simulink model "simpleMicrogrid_v3_0_18a"  (R2018a)
settings: Solver=VariableStepAuto  StartTime=0.0  StopTime=30  RelTol=1e-3
undefined symbols (not defined in the file or in its folder): Ion, Lithium
libraries: simulink x21, spsSeriesRLCBranchLib x13, spsIdealSwitchLib x10, spsMosfetLib x8, spsPWMGeneratorDCDCLib x6, spsVoltageMeasurementLib x5, spsThreePhaseSeriesRLCLoadLib x3, spsThreePhaseSeriesRLCBranchLib x3, spsThreePhaseDynamicLoadLib x3, spsGroundLib x2, spsThreePhaseVIMeasurementLib x2, spsUniversalBridgeLib x2
(part 1 of 2)
settings Model: SimulationMode=accelerator  Creator=jakub  LastModifiedBy=mluser
settings DataIOCC: ReturnWorkspaceOutputs=on
settings SFSimCC: SimUseLocalCustomCode=on
settings RTWCC: RTWUseLocalCustomCode=on

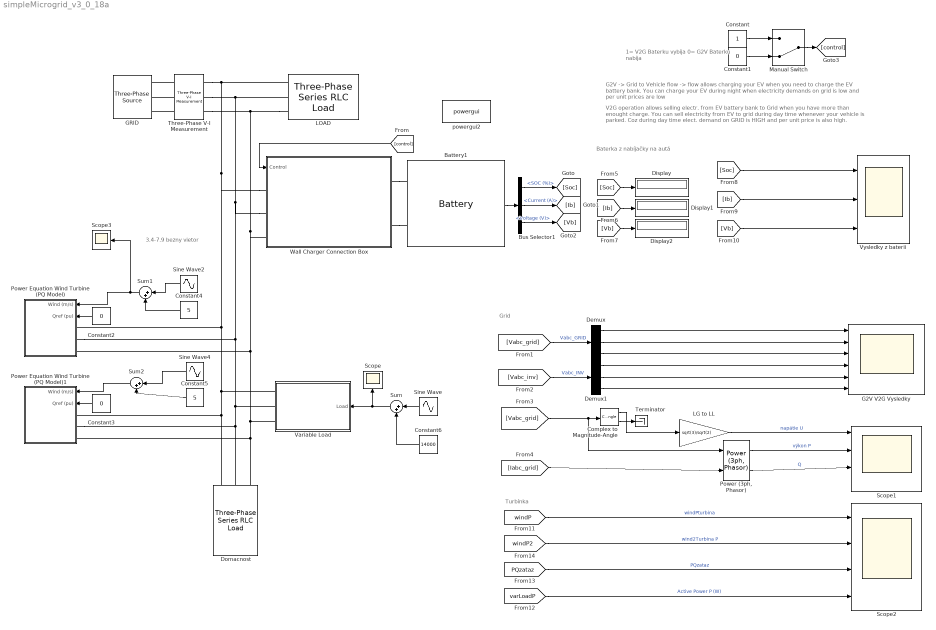
== system simpleMicrogrid_v3_0_18a ==
  note: 3.4-7.9 bezny vietor
  note: Baterka z nabíjačky na autá
  note: Turbínka
  note: Grid
  note: 1= V2G Baterku vybíja
      | 0= G2V Baterku nabíja
  note: G2V -> Grid to Vehicle flow -> flow allows charging your EV when you need to charge the EV battery bank. You can charge your EV during night when electricity demands on grid is low and per unit prices are low
  note: V2G operation allows selling electr. from EV battery bank to Grid when you have more than enought charge. You can sell electricity from EV to grid during day time whenever your vehicle is parked. Coz during day time elect. demand on GRID is HIGH and per unit price is also high.
  Battery1 : spsBatteryLib/Battery  BatType=Lithium-Ion  ShowTempParam=off  ThermalPreset=no  ShowAgeParam=off  NomV=230  NomQ=100  SOC=60  Batt_Tr=1e-3  PresetModel=on  MaxQ=100  MinV=172.5  FullV=267.717  Dis_rate=43.4783  R=0.023  Normal_OP=90.4348  expZone="[248.4887      4.913043]"  current=[6.5 13 32.5]  Units=Time  Tci=20  NomT=20  T2=-30  MaxQ2=4.8  FullV2=7.1  Normal_OP2=5.655  expZone2="[6.58           1]"  Rca=0.6  ti=2000  Dp=0  Neq0=0  Tsim=1e6  Ta1=25  Qeol=5.4*0.9  Reol=0.013333*1.2  Char_age=[2.3478, 3]  Dis_age=[2.3478, 10]  N1=1500  N2=10500  N3=1000  N4=1400  Ta2=45  N5=950
  Bus Selector1 : BusSelector  OutputSignals=SOC (%),Current (A),Voltage (V)
  Complex to Magnitude-Angle : ComplexToMagnitudeAngle
  Constant : Constant
  Constant1 : Constant  Value=0
  Constant2 : Constant  Value=0
  Constant3 : Constant  Value=0
  Constant4 : Constant  Value=5
  Constant5 : Constant  Value=5
  Constant6 : Constant  Value=14000
  Demux : Demux  Outputs=3
  Demux1 : Demux  Outputs=3
  Display : Display
  Display1 : Display
  Display2 : Display
  Domacnost : spsThreePhaseSeriesRLCLoadLib/Three-Phase Series RLC Load  LConnTagsString=A|B|C  Configuration=Y (grounded)  NominalVoltage=380  Vabc=[1e3 1e3 1e3]  Vabcp=[1e3 1e3 1e3]  NominalFrequency=50  UnbalancedPower=off  ActivePower=10e3  InductivePower=0  CapacitivePower=0  Pabc=[10e3 9e3 11e3]  QLabc=[100 90 110]  QCabc=[100 90 110]  Pabcp=[10e3 9e3 11e3]  QLabcp=[100 90 110]  QCabcp=[100 90 110]  Measurements=None  LoadType=constant Z
  G2V V2G Vysledky : Scope  NumInputPorts=6
  GRID : spsThreePhaseSourceLib/Three-Phase Source  InternalConnection=Yg  VoltagePhases=off  Voltage=380  PhaseAngle=0  Voltage_phases=[25e3 25e3 25e3]/sqrt(3)  PhaseAngles_phases=[0 -120 +120]  Frequency=50  NonIdealSource=on  SpecifyImpedance=on  Resistance=0.8929  Inductance=16.58e-3  ShortCircuitLevel=100e6  BaseVoltage=380  XRratio=7  BusType=swing  Pref=10e3  Qref=0  Prefabc=[10e3, 10e3, 10e3]  Qrefabc=[0, 0, 0]  Qmin=-inf  Qmax=inf
  LG to LL : Gain  Gain=sqrt(3)/sqrt(2)
  LOAD : spsThreePhaseSeriesRLCLoadLib/Three-Phase Series RLC Load  LConnTagsString=A|B|C  Configuration=Y (grounded)  NominalVoltage=380  Vabc=[1e3 1e3 1e3]  Vabcp=[1e3 1e3 1e3]  NominalFrequency=50  UnbalancedPower=off  ActivePower=10e3  InductivePower=0  CapacitivePower=0  Pabc=[10e3 9e3 11e3]  QLabc=[100 90 110]  QCabc=[100 90 110]  Pabcp=[10e3 9e3 11e3]  QLabcp=[100 90 110]  QCabcp=[100 90 110]  Measurements=None  LoadType=constant Z
  Manual Switch : ManualSwitch  CurrentSetting=0
  "Power (3ph, Phasor)" : spsPower3phPhasorLib/Power (3ph, Phasor)
      settings: SourceProductBaseCode=PS
  Power Equation Wind Turbine (PQ Model) : Subsystem  AncestorBlock=|  mask{Unom=15, Umax=25, Umin=5, Pselect=Simple Cubic Power, rp=5, Cp=16/27, rho=1.225, Pnom=500e3, Uvec=[1:1:30], Pvec=[0,0,0,0,21359.3750000000,58193.5000000000,104316.125000000,157104.500000000,213935.875000000,272187.500000000,329236.625000000,382460.500000000,429236.375000000,466941.500000000,492953.125000000,500000,500000,500000,500000,500000,500000,500000,500000,500000,500000,0,0,0,0,0], Tp=0.1, Tq=1, ReactP=30}
      | exampleMicrogridLibrary/Power Equation
      | Wind Turbine
      | (PQ Model)
      mask prompts: Unom "Nominal Wind Speed [m/s]"; Umax "Maximum Operating Wind [m/s]"; Umin "Minimum Operating Wind [m/s]"; Pselect "Wind Turbine Power Method"; rp "Blade Radius, r [m]"; Cp "Performance Coefficient, Cp"; rho "Air Density, rho [kg/m^3]"; Pnom "Nominal Power, [W]"; Uvec "Wind Vec [m/s]"; Pvec "Power Vec [W]"; Tp "Active Power Dynamics, Tp [s]"; Tq "Reactive Power Dynamics, Tq [s]"; ReactP "Reactive Power Percentage [%]"
      mask help:
      | Simple Wind Turbine that serves as an Active and Reactive Power Source depending on the Wind Power Curve.
      |
      | The Wind Turbine Power Curve can be defined by:
      | - Dimentions of the wind turbine
      | - Simple cubic power curve
      | - Look-up vector from a wind turbine data sheet.
      mask init:
      | A = pi*rp^2;
      | 
      | if Pselect == 1,
      |     Pmax = 1/2*rho*Cp*A*Umax^3;
      | elseif Pselect == 2,
      |     Pmax = Pnom;
      | else
      |     Pmax = max(Pvec);
      | end
      | Qmax = ReactP/100*Pmax;
      mask TypeOptions Pselect: Using Properties | Simple Cubic Power | Look-up Fit
      mask DialogControl Container4 Prompt: General
      mask DialogControl Container9 Prompt: Dimensions
      mask DialogControl Container12 Prompt: Cubic
      mask DialogControl Container7 Prompt: Lookup
      mask DialogControl Container8 Prompt: Dynamics
  Power Equation Wind Turbine (PQ Model)1 : Subsystem  AncestorBlock=|  mask{Unom=15, Umax=25, Umin=5, Pselect=Simple Cubic Power, rp=5, Cp=16/27, rho=1.225, Pnom=500e3, Uvec=[1:1:30], Pvec=[0,0,0,0,21359.3750000000,58193.5000000000,104316.125000000,157104.500000000,213935.875000000,272187.500000000,329236.625000000,382460.500000000,429236.375000000,466941.500000000,492953.125000000,500000,500000,500000,500000,500000,500000,500000,500000,500000,500000,0,0,0,0,0], Tp=0.1, Tq=1, ReactP=30}
      | exampleMicrogridLibrary/Power Equation
      | Wind Turbine
      | (PQ Model)
      mask prompts: Unom "Nominal Wind Speed [m/s]"; Umax "Maximum Operating Wind [m/s]"; Umin "Minimum Operating Wind [m/s]"; Pselect "Wind Turbine Power Method"; rp "Blade Radius, r [m]"; Cp "Performance Coefficient, Cp"; rho "Air Density, rho [kg/m^3]"; Pnom "Nominal Power, [W]"; Uvec "Wind Vec [m/s]"; Pvec "Power Vec [W]"; Tp "Active Power Dynamics, Tp [s]"; Tq "Reactive Power Dynamics, Tq [s]"; ReactP "Reactive Power Percentage [%]"
      mask help:
      | Simple Wind Turbine that serves as an Active and Reactive Power Source depending on the Wind Power Curve.
      |
      | The Wind Turbine Power Curve can be defined by:
      | - Dimentions of the wind turbine
      | - Simple cubic power curve
      | - Look-up vector from a wind turbine data sheet.
      mask init:
      | A = pi*rp^2;
      | 
      | if Pselect == 1,
      |     Pmax = 1/2*rho*Cp*A*Umax^3;
      | elseif Pselect == 2,
      |     Pmax = Pnom;
      | else
      |     Pmax = max(Pvec);
      | end
      | Qmax = ReactP/100*Pmax;
      mask TypeOptions Pselect: Using Properties | Simple Cubic Power | Look-up Fit
      mask DialogControl Container4 Prompt: General
      mask DialogControl Container9 Prompt: Dimensions
      mask DialogControl Container12 Prompt: Cubic
      mask DialogControl Container7 Prompt: Lookup
      mask DialogControl Container8 Prompt: Dynamics
  Scope : Scope
  Scope1 : Scope  NumInputPorts=4
  Scope2 : Scope  NumInputPorts=4
  Scope3 : Scope
  Sine Wave : Sin  Amplitude=11000  Frequency=1/2  SampleTime=0
  Sine Wave2 : Sin  Amplitude=1.2  Frequency=1/2  SampleTime=0
  Sine Wave4 : Sin  Amplitude=1.2  Frequency=1/2  SampleTime=0
  Sum : Sum  Inputs=|++
  Sum1 : Sum  Inputs=|++
  Sum2 : Sum  Inputs=|++
  Terminator : Terminator
  Three-Phase V-I Measurement : spsThreePhaseVIMeasurementLib/Three-Phase V-I Measurement  VoltageMeasurement=phase-to-phase  SetLabelV=on  LabelV=Vabc_grid  Vpu=off  VpuLL=off  CurrentMeasurement=yes  SetLabelI=on  LabelI=Iabc_grid  Ipu=off  Pbase=100e6  Vbase=500e3  OutputType=Complex  PhasorSimulation=off  PSBequivalent=0
  Variable Load : Subsystem  mask(Variable Load (PQ Model)){Vn=4500, Fn=60, PF=0.8, Load0=25e4}
      mask prompts: Vn "Nominal L-L Voltage [Vrms]"; Fn "Nominal Frequency [Hz]"; PF "Power Factor [0 to 1]"; Load0 "Initial Load [W]"
      mask help:
      | The Variable Load block is a lumped approximation for a distribution feeder. For non-unity power factor loads, the input (active power) is scaled accordingly to generate a desired load.
      |
      | Note: The initial input load must be specified for use for Load Flow analysis.
      mask init:
      | P0 = Load0;
      | Q0 = Load0*sqrt(1/PF-1);
      mask Display:
      | image(imread('Residential.jpg'))
      | color('white')
      | port_label('input',1,'Load')
      | port_label('Rconn',1,'A')
      | port_label('Rconn',2,'B')
      | port_label('Rconn',3,'C')
  Vysledky z baterii : Scope  NumInputPorts=3
  Wall Charger Connection Box : Subsystem
      mask help:
      | This block contains :
      | ->Connection  control
      | ->DC-AC/AC-DC converter
      | ->Buck-boost  converter
      | ->DC-DC converter with B.controller
      | ->Battery switching control
      mask Display: image('dipolar.jpg'); % Use "Edit Image" on toolstrip to change.
  powergui2 : spspowerguiLib/powergui  Priority=1  SimulationMode=Discrete  SampleTime=5e-6  frequency=60  Iterations=50  frequencyindice=0  Pbase=100e6  ErrMax=1e-4  UnitsV=kV  UnitsW=MW  buscounter=0  FunctionMessages=off  echomessages=off  EnableUseOfTLC=off  CurrentSourceSwitches=off  DisableSnubberDevices=off  DisableRonSwitches=off  DisableVfSwitches=off  DisplayEquations=off  AutomaticDiscreteSolvers=off  SolverType=Tustin/Backward Euler (TBE)  Interpol=off  ExternalGateDelay=off  methode=off  Ts=100  x0status=blocks  SPID=on  SwTol=0  HookPort=off  NonlinearTolerance=1e-4  nMaxIteration=100  ContinueOnMaxIteration=off  RestoreLinks=warning  ResistiveCurrentMeasurement=off  Frange=[0:2:500]  Ylog=off  Xlog=on  ShowGrid=off  save=off  variable=ZData  structure=0  ZoomFFT=off  StartTime=0.0  cycles=1  DisplayStyle=1  fundamental=60  FreqAxis=off  MaxFrequency=1000  frequencyindicesteady=1  RmsSteady=1  display=off
  wires:
  Demux1/3 -> G2V V2G Vysledky/6
  Constant1/1 -> Manual Switch/2
  [Soc] -> Vysledky z baterii/1
  [Soc] -> Display/1
  [Vabc_grid] -> Demux/1  "Vabc_GRID"
  [Vabc_inv] -> Demux1/1  "Vabc_INV"
  Demux/1 -> G2V V2G Vysledky/1
  Demux1/1 -> G2V V2G Vysledky/4
  [Vb] -> Vysledky z baterii/3
  Bus Selector1/2 -> [Ib]  "<Current (A)>"
  [control] -> Wall Charger Connection Box/1(Control)
  Bus Selector1/3 -> [Vb]  "<Voltage (V)>"
  Bus Selector1/1 -> [Soc]  "<SOC (%)>"
  [Vb] -> Display2/1
  Battery1/1 -> Bus Selector1/1
  Demux/2 -> G2V V2G Vysledky/2
  [Ib] -> Vysledky z baterii/2
  [Ib] -> Display1/1
  Demux/3 -> G2V V2G Vysledky/3
  Manual Switch/1 -> [control]
  Constant/1 -> Manual Switch/1
  Demux1/2 -> G2V V2G Vysledky/5
  Sine Wave/1 -> Sum/1
  Constant6/1 -> Sum/2
  Sum/1 -> Scope/1, Variable Load/1(Load)
  Constant2/1 -> Power Equation Wind Turbine (PQ Model)/2(Qref (pu))
  LG to LL/1 -> Scope1/1  "napätie U"
  [Vabc_grid] -> "Power (3ph, Phasor)"/1, Complex to Magnitude-Angle/1
  [Iabc_grid] -> "Power (3ph, Phasor)"/2
  "Power (3ph, Phasor)"/1 -> Scope1/2  "výkon P"
  "Power (3ph, Phasor)"/2 -> Scope1/3  "Q"
  Complex to Magnitude-Angle/1 -> LG to LL/1
  Complex to Magnitude-Angle/2 -> Terminator/1
  Sum1/1 -> Scope3/1, Power Equation Wind Turbine (PQ Model)/1(Wind (m/s))
  [windP] -> Scope2/1  "windPturbina"
  [PQzataz] -> Scope2/3  "PQzataz"
  [varLoadP] -> Scope2/4  "Active Power P (W)"
  Sum2/1 -> Power Equation Wind Turbine (PQ Model)1/1(Wind (m/s))
  Constant3/1 -> Power Equation Wind Turbine (PQ Model)1/2(Qref (pu))
  [windP2] -> Scope2/2  "wind2Turbina P"
  Sine Wave2/1 -> Sum1/1
  Constant4/1 -> Sum1/2
  Constant5/1 -> Sum2/2
  Sine Wave4/1 -> Sum2/1
  connections:
  LOAD/LConn3 -- Three-Phase V-I Measurement/RConn3 -- Domacnost/LConn3 -- Power Equation Wind Turbine (PQ Model)1/LConn3 -- Variable Load/RConn3 -- Power Equation Wind Turbine (PQ Model)/LConn3 -- Wall Charger Connection Box/LConn3
  Wall Charger Connection Box/LConn1 -- Power Equation Wind Turbine (PQ Model)1/LConn1 -- Domacnost/LConn1 -- Variable Load/RConn1 -- Power Equation Wind Turbine (PQ Model)/LConn1 -- Three-Phase V-I Measurement/RConn1 -- LOAD/LConn1
  Wall Charger Connection Box/LConn2 -- Power Equation Wind Turbine (PQ Model)1/LConn2 -- Domacnost/LConn2 -- Variable Load/RConn2 -- Power Equation Wind Turbine (PQ Model)/LConn2 -- LOAD/LConn2 -- Three-Phase V-I Measurement/RConn2
  Three-Phase V-I Measurement/LConn3 -- GRID/RConn3
  Wall Charger Connection Box/RConn2 -- Battery1/LConn1
  Wall Charger Connection Box/RConn1 -- Battery1/LConn2
  Three-Phase V-I Measurement/LConn1 -- GRID/RConn1
  Three-Phase V-I Measurement/LConn2 -- GRID/RConn2

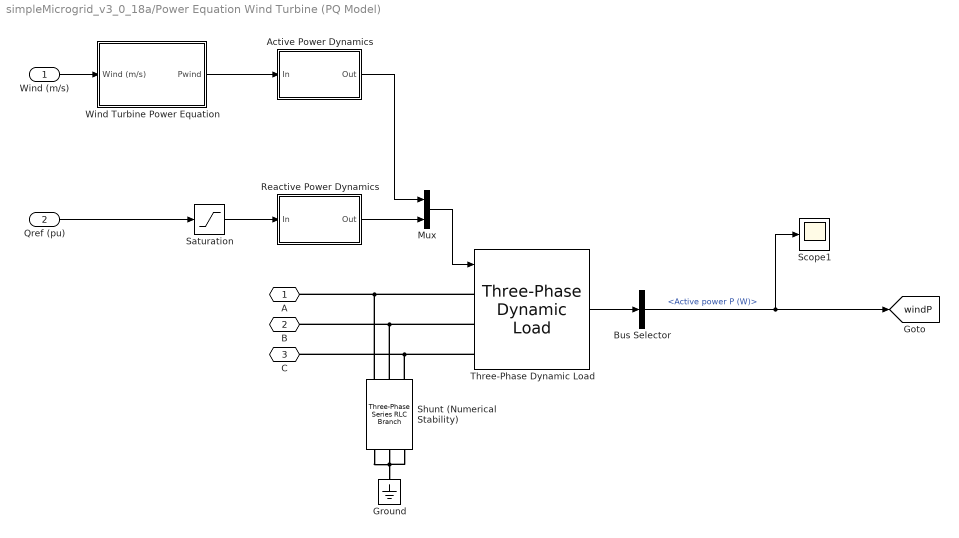
== system simpleMicrogrid_v3_0_18a/Power Equation Wind Turbine (PQ Model) ==
  Wind (m/s) : Inport
  Qref (pu) : Inport  Port=2
  Active Power Dynamics : Subsystem  VariantControl=T6NotZero
      mask Display: disp('1 / (1 + s T_P)','texmode','on');
  Bus Selector : BusSelector  OutputSignals=Active power P (W)
  Ground : spsGroundLib/Ground  LConnTagsString=a
  Mux : Mux  Inputs=2
  Reactive Power Dynamics : Subsystem  VariantControl=T6NotZero
      mask Display: disp('1 / (1 + s T_Q)','texmode','on');
  Saturation : Saturate  UpperLimit=Qmax  LowerLimit=-Qmax
  Scope1 : Scope
  Shunt (Numerical Stability) : spsThreePhaseSeriesRLCBranchLib/Three-Phase Series RLC Branch  LConnTagsString=A|B|C  RConnTagsString=A|B|C  BranchType=R  Resistance=1e9  Inductance=1e-3  Capacitance=1e-6  Measurements=None
  Three-Phase Dynamic Load : spsThreePhaseDynamicLoadLib/Three-Phase Dynamic Load  NominalVoltage=[5000 60]  ActiveReactivePowers=[50e6 25e6]  PositiveSequence=[0.994 -11.8]  ExternalControl=on  NpNq=[1.3 2]  TimeConstants="[0  0  0  0]"  MinimumVoltage=0.7  Tfilter=1e-4  LoadFlowParameters=[4,0,0,0,0]
      settings: SourceProductBaseCode=PS
  Wind Turbine Power Equation : Subsystem
  A : PMIOPort  Side=Left
  B : PMIOPort  Port=2  Side=Left
  C : PMIOPort  Port=3  Side=Left
  tag scope: windP=global
  wires:
  Qref (pu)/1 -> Saturation/1
  Saturation/1 -> Reactive Power Dynamics/1(In)
  Reactive Power Dynamics/1(Out) -> Mux/2
  Active Power Dynamics/1(Out) -> Mux/1
  Mux/1 -> Three-Phase Dynamic Load/1
  Wind Turbine Power Equation/1(Pwind) -> Active Power Dynamics/1(In)
  Wind (m/s)/1 -> Wind Turbine Power Equation/1(Wind (m/s))
  Bus Selector/1 -> Scope1/1, [windP]  "<Active power P (W)>"
  Three-Phase Dynamic Load/1 -> Bus Selector/1
  connections:
  Ground/LConn1 -- Shunt (Numerical Stability)/RConn1 -- Shunt (Numerical Stability)/RConn2 -- Shunt (Numerical Stability)/RConn3
  Shunt (Numerical Stability)/LConn1 -- Three-Phase Dynamic Load/LConn1 -- A/RConn1
  Shunt (Numerical Stability)/LConn3 -- Three-Phase Dynamic Load/LConn3 -- C/RConn1
  Shunt (Numerical Stability)/LConn2 -- Three-Phase Dynamic Load/LConn2 -- B/RConn1

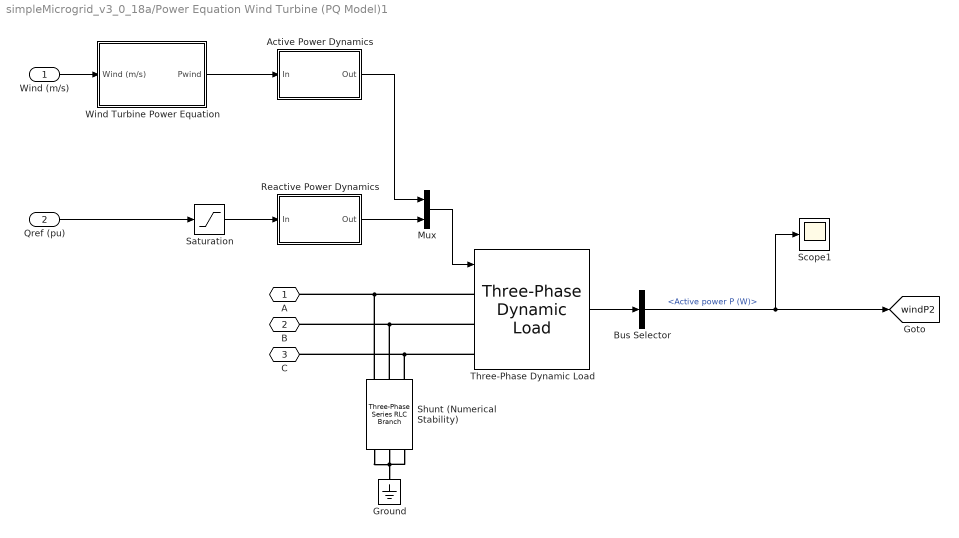
== system simpleMicrogrid_v3_0_18a/Power Equation Wind Turbine (PQ Model)1 ==
  Wind (m/s) : Inport
  Qref (pu) : Inport  Port=2
  Active Power Dynamics : Subsystem  VariantControl=T6NotZero
      mask Display: disp('1 / (1 + s T_P)','texmode','on');
  Bus Selector : BusSelector  OutputSignals=Active power P (W)
  Ground : spsGroundLib/Ground  LConnTagsString=a
  Mux : Mux  Inputs=2
  Reactive Power Dynamics : Subsystem  VariantControl=T6NotZero
      mask Display: disp('1 / (1 + s T_Q)','texmode','on');
  Saturation : Saturate  UpperLimit=Qmax  LowerLimit=-Qmax
  Scope1 : Scope
  Shunt (Numerical Stability) : spsThreePhaseSeriesRLCBranchLib/Three-Phase Series RLC Branch  LConnTagsString=A|B|C  RConnTagsString=A|B|C  BranchType=R  Resistance=1e9  Inductance=1e-3  Capacitance=1e-6  Measurements=None
  Three-Phase Dynamic Load : spsThreePhaseDynamicLoadLib/Three-Phase Dynamic Load  NominalVoltage=[5000 60]  ActiveReactivePowers=[50e6 25e6]  PositiveSequence=[0.994 -11.8]  ExternalControl=on  NpNq=[1.3 2]  TimeConstants="[0  0  0  0]"  MinimumVoltage=0.7  Tfilter=1e-4  LoadFlowParameters=[4,0,0,0,0]
      settings: SourceProductBaseCode=PS
  Wind Turbine Power Equation : Subsystem
  A : PMIOPort  Side=Left
  B : PMIOPort  Port=2  Side=Left
  C : PMIOPort  Port=3  Side=Left
  tag scope: windP2=global
  wires:
  Qref (pu)/1 -> Saturation/1
  Saturation/1 -> Reactive Power Dynamics/1(In)
  Reactive Power Dynamics/1(Out) -> Mux/2
  Active Power Dynamics/1(Out) -> Mux/1
  Mux/1 -> Three-Phase Dynamic Load/1
  Wind Turbine Power Equation/1(Pwind) -> Active Power Dynamics/1(In)
  Wind (m/s)/1 -> Wind Turbine Power Equation/1(Wind (m/s))
  Bus Selector/1 -> Scope1/1, [windP2]  "<Active power P (W)>"
  Three-Phase Dynamic Load/1 -> Bus Selector/1
  connections:
  Ground/LConn1 -- Shunt (Numerical Stability)/RConn1 -- Shunt (Numerical Stability)/RConn2 -- Shunt (Numerical Stability)/RConn3
  Shunt (Numerical Stability)/LConn1 -- Three-Phase Dynamic Load/LConn1 -- A/RConn1
  Shunt (Numerical Stability)/LConn3 -- Three-Phase Dynamic Load/LConn3 -- C/RConn1
  Shunt (Numerical Stability)/LConn2 -- Three-Phase Dynamic Load/LConn2 -- B/RConn1

== system simpleMicrogrid_v3_0_18a/Variable Load ==
  Load : Inport
  Bus Selector : BusSelector  OutputSignals=Active power P (W)
  Dynamic Load Control : Subsystem
  Scope : Scope
  Simple Three-Phase Load : spsThreePhaseDynamicLoadLib/Three-Phase Dynamic Load  NominalVoltage=[Vn Fn]  ActiveReactivePowers=[200000 45883.1]  PositiveSequence=[0.999962 -0.018842]  ExternalControl=on  NpNq=[1.3 2]  TimeConstants="[0  0  0  0]"  MinimumVoltage=0.7  Tfilter=1e-2  LoadFlowParameters=[4,0,0,0,0]
      settings: SourceProductBaseCode=PS
  A : PMIOPort  Side=Right
  B : PMIOPort  Port=2  Side=Right
  C : PMIOPort  Port=3  Side=Right
  tag scope: PQzataz=global, varLoadP=global
  wires:
  Simple Three-Phase Load/1 -> Bus Selector/1
  Load/1 -> Dynamic Load Control/1(P0)
  Dynamic Load Control/1(PQ) -> [PQzataz], Scope/1, Simple Three-Phase Load/1
  Bus Selector/1 -> [varLoadP]  "<Active power P (W)>"
  connections:
  Simple Three-Phase Load/LConn1 -- A/RConn1
  Simple Three-Phase Load/LConn3 -- C/RConn1
  Simple Three-Phase Load/LConn2 -- B/RConn1

== system simpleMicrogrid_v3_0_18a/Wall Charger Connection Box ==
  Control : Inport
  Battery Switching Control : Subsystem
  Buck-Boost Converter : Subsystem
      mask help:
      | A buck boost application is best explained in terms of a battery powered system.
      | The “boost” portion of the buck-boost converter is used to make the input voltage produce
      | an output voltage that is greater than the input voltage.
      | This allows the max voltage to charge the system as quick as possible.
  Connection Control : Subsystem
  DC-AC / AC-DC Converter : Subsystem
  DC-DC Converter with Battery Controller : Subsystem
  GRID R : PMIOPort  Side=Left
  GRID Y : PMIOPort  Port=2  Side=Left
  GRID B : PMIOPort  Port=3  Side=Left
  Vehicle - : PMIOPort  Port=4  Side=Right
  Vehicle + : PMIOPort  Port=5  Side=Right
  wires:
  Control/1 -> Battery Switching Control/1(control), Connection Control/1(control)
  connections:
  Battery Switching Control/RConn6 -- Vehicle +/RConn1
  Battery Switching Control/RConn5 -- Vehicle -/RConn1
  Battery Switching Control/RConn4 -- DC-DC Converter with Battery Controller/RConn5
  DC-DC Converter with Battery Controller/RConn6 -- Battery Switching Control/RConn3
  Battery Switching Control/RConn1 -- DC-DC Converter with Battery Controller/RConn3
  Battery Switching Control/RConn2 -- DC-DC Converter with Battery Controller/RConn4
  DC-DC Converter with Battery Controller/RConn1 -- Buck-Boost Converter/RConn7
  DC-DC Converter with Battery Controller/RConn2 -- Buck-Boost Converter/RConn8
  DC-DC Converter with Battery Controller/LConn2 -- Buck-Boost Converter/RConn6
  DC-DC Converter with Battery Controller/LConn1 -- Buck-Boost Converter/RConn5
  Buck-Boost Converter/RConn4 -- DC-AC / AC-DC Converter/RConn10
  Buck-Boost Converter/RConn3 -- DC-AC / AC-DC Converter/RConn9
  Buck-Boost Converter/RConn2 -- DC-AC / AC-DC Converter/RConn8
  DC-AC / AC-DC Converter/RConn7 -- Buck-Boost Converter/RConn1
  DC-AC / AC-DC Converter/RConn6 -- Connection Control/RConn6
  Connection Control/RConn5 -- DC-AC / AC-DC Converter/RConn5
  Connection Control/RConn4 -- DC-AC / AC-DC Converter/RConn4
  DC-AC / AC-DC Converter/RConn3 -- Connection Control/RConn3
  Connection Control/RConn2 -- DC-AC / AC-DC Converter/RConn2
  Connection Control/RConn1 -- DC-AC / AC-DC Converter/RConn1
  GRID R/RConn1 -- Connection Control/LConn1
  GRID Y/RConn1 -- Connection Control/LConn2
  GRID B/RConn1 -- Connection Control/LConn3

== system simpleMicrogrid_v3_0_18a/Power Equation Wind Turbine (PQ Model)/Active Power Dynamics ==
  In : Inport
  1/Tp : Gain  Gain=1/Tp
  Integrator : Integrator
  Sum : Sum  Inputs=|+-
  Out : Outport  VectorParamsAs1DForOutWhenUnconnected=off
  wires:
  Sum/1 -> 1/Tp/1
  1/Tp/1 -> Integrator/1
  In/1 -> Sum/1
  Integrator/1 -> Sum/2, Out/1

== system simpleMicrogrid_v3_0_18a/Power Equation Wind Turbine (PQ Model)/Reactive Power Dynamics ==
  In : Inport
  1/Tq : Gain  Gain=1/Tq
  Integrator : Integrator
  Sum : Sum  Inputs=|+-
  Out : Outport  VectorParamsAs1DForOutWhenUnconnected=off
  wires:
  Integrator/1 -> Out/1, Sum/2
  In/1 -> Sum/1
  1/Tq/1 -> Integrator/1
  Sum/1 -> 1/Tq/1

== system simpleMicrogrid_v3_0_18a/Power Equation Wind Turbine (PQ Model)/Wind Turbine Power Equation ==
  Wind (m/s) : Inport
  Constant : Constant  Value=Pselect
  Cubic Power with Cutoff : Subsystem
  Manufacturer Fit : Lookup_n-D  NumberOfTableDimensions=1  BreakpointsForDimension1=Uvec  Table=Pvec  ExtrapMethod=Clip  InternalRulePriority=Speed  RndMeth=Simplest  InputSameDT=on
  Multiport Switch : MultiPortSwitch
  Saturation : Saturate  UpperLimit=inf  LowerLimit=0  ZeroCross=off
      settings: AttributesFormatString=|
      | %<UpperLimit>
      | %<LowerLimit>
  Wind Turbine Properties : Subsystem
  Pwind : Outport  VectorParamsAs1DForOutWhenUnconnected=off
  wires:
  Wind (m/s)/1 -> Saturation/1
  Multiport Switch/1 -> Pwind/1
  Constant/1 -> Multiport Switch/1
  Saturation/1 -> Wind Turbine Properties/1(Wind (m/s)), Manufacturer Fit/1, Cubic Power with Cutoff/1(Wind (m/s))
  Cubic Power with Cutoff/1(Pwind) -> Multiport Switch/3
  Manufacturer Fit/1 -> Multiport Switch/4
  Wind Turbine Properties/1(Pwind) -> Multiport Switch/2

== system simpleMicrogrid_v3_0_18a/Power Equation Wind Turbine (PQ Model)1/Active Power Dynamics ==
  In : Inport
  1/Tp : Gain  Gain=1/Tp
  Integrator : Integrator
  Sum : Sum  Inputs=|+-
  Out : Outport  VectorParamsAs1DForOutWhenUnconnected=off
  wires:
  Sum/1 -> 1/Tp/1
  1/Tp/1 -> Integrator/1
  In/1 -> Sum/1
  Integrator/1 -> Sum/2, Out/1

== system simpleMicrogrid_v3_0_18a/Power Equation Wind Turbine (PQ Model)1/Reactive Power Dynamics ==
  In : Inport
  1/Tq : Gain  Gain=1/Tq
  Integrator : Integrator
  Sum : Sum  Inputs=|+-
  Out : Outport  VectorParamsAs1DForOutWhenUnconnected=off
  wires:
  Integrator/1 -> Out/1, Sum/2
  In/1 -> Sum/1
  1/Tq/1 -> Integrator/1
  Sum/1 -> 1/Tq/1

== system simpleMicrogrid_v3_0_18a/Power Equation Wind Turbine (PQ Model)1/Wind Turbine Power Equation ==
  Wind (m/s) : Inport
  Constant : Constant  Value=Pselect
  Cubic Power with Cutoff : Subsystem
  Manufacturer Fit : Lookup_n-D  NumberOfTableDimensions=1  BreakpointsForDimension1=Uvec  Table=Pvec  ExtrapMethod=Clip  InternalRulePriority=Speed  RndMeth=Simplest  InputSameDT=on
  Multiport Switch : MultiPortSwitch
  Saturation : Saturate  UpperLimit=inf  LowerLimit=0  ZeroCross=off
      settings: AttributesFormatString=|
      | %<UpperLimit>
      | %<LowerLimit>
  Wind Turbine Properties : Subsystem
  Pwind : Outport  VectorParamsAs1DForOutWhenUnconnected=off
  wires:
  Wind (m/s)/1 -> Saturation/1
  Multiport Switch/1 -> Pwind/1
  Constant/1 -> Multiport Switch/1
  Saturation/1 -> Wind Turbine Properties/1(Wind (m/s)), Manufacturer Fit/1, Cubic Power with Cutoff/1(Wind (m/s))
  Cubic Power with Cutoff/1(Pwind) -> Multiport Switch/3
  Manufacturer Fit/1 -> Multiport Switch/4
  Wind Turbine Properties/1(Pwind) -> Multiport Switch/2

== system simpleMicrogrid_v3_0_18a/Variable Load/Dynamic Load Control ==
  P0 : Inport
  Fcn : Fcn  Expr=sqrt(1/u(1)-1)
  Mux : Mux  Inputs=2
  Product : Product
  Summer1 : Constant  Value=PF
  PQ : Outport  VectorParamsAs1DForOutWhenUnconnected=off
  wires:
  Summer1/1 -> Fcn/1
  Fcn/1 -> Product/2
  P0/1 -> Product/1, Mux/1
  Mux/1 -> PQ/1
  Product/1 -> Mux/2  "Qo"

== system simpleMicrogrid_v3_0_18a/Wall Charger Connection Box/Battery Switching Control ==
  control : Inport
  Ideal Switch{,1..3} (4 alike) : spsIdealSwitchLib/Ideal Switch  Ron=0.001  Lon=0  IC=0  Rs=1e5  Cs=inf  Measurements=off
  NOT : Logic  Operator=NOT  IconShape=distinctive  AllPortsSameDT=off  OutDataTypeStr=boolean
  discharge + : PMIOPort  Side=Right
  discharge - : PMIOPort  Port=2  Side=Right
  charge + : PMIOPort  Port=3  Side=Right
  charge - : PMIOPort  Port=4  Side=Right
  Battery- : PMIOPort  Port=5  Side=Right
  Battery+ : PMIOPort  Port=6  Side=Right
  wires:
  control/1 -> NOT/1, Ideal Switch1/1, Ideal Switch/1
  NOT/1 -> Ideal Switch3/1, Ideal Switch2/1
  connections:
  Ideal Switch/RConn1 -- discharge +/RConn1
  discharge -/RConn1 -- Ideal Switch1/RConn1
  Ideal Switch2/RConn1 -- charge +/RConn1
  charge -/RConn1 -- Ideal Switch3/RConn1
  Battery+/RConn1 -- Ideal Switch2/LConn1 -- Ideal Switch/LConn1
  Ideal Switch1/LConn1 -- Ideal Switch3/LConn1 -- Battery-/RConn1

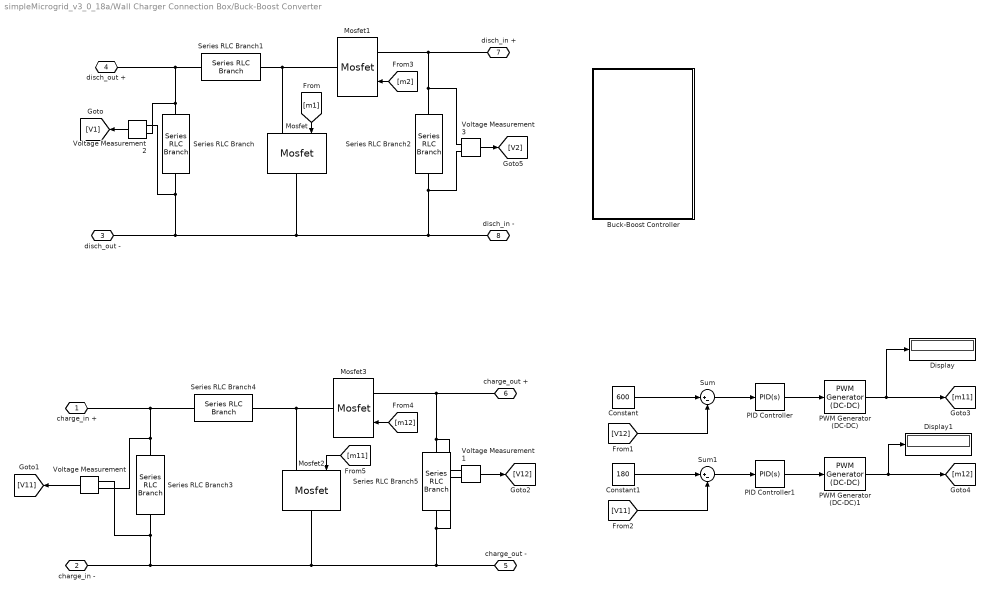
== system simpleMicrogrid_v3_0_18a/Wall Charger Connection Box/Buck-Boost Converter ==
  Buck-Boost Controller : Subsystem
  Constant : Constant  Value=600
  Constant1 : Constant  Value=180
  Display : Display
  Display1 : Display
  Mosfet{,1..3} (4 alike) : spsMosfetLib/Mosfet  Ron=0.1  Lon=0  Rd=0.01  Vfd=0  IC=0  Rs=1e5  Cs=inf  Measurements=off
  PID Controller : simulink/Continuous/PID Controller  Controller=PID  Form=Parallel  TimeDomain=Continuous-time  SampleTime=-1  IntegratorMethod=Forward Euler  ControllerParametersSource=internal  P=0  I=7  D=0  UseFilter=on  N=100  TunerSelectOption=Transfer Function Based (PID Tuner App)  InitialConditionSource=internal  InitialConditionForIntegrator=0  InitialConditionForFilter=0  DifferentiatorICPrevScaledInput=0  ExternalReset=none  TrackingMode=off  Kt=1  LimitOutput=off  UpperSaturationLimit=inf  LowerSaturationLimit=-inf  LinearizeAsGain=on  AntiWindupMode=none  Kb=1  POutMin=[]  POutMax=[]  IOutMin=[]  IOutMax=[]  DOutMin=[]  DOutMax=[]  NOutMin=[]  NOutMax=[]  SumOutMin=[]  SumOutMax=[]  SaturationOutMin=[]  SaturationOutMax=[]  PParamMin=[]  PParamMax=[]  IParamMin=[]  IParamMax=[]  DParamMin=[]  DParamMax=[]  NParamMin=[]  NParamMax=[]  KbParamMin=[]  KbParamMax=[]  KtParamMin=[]  KtParamMax=[]  KbOutMin=[]  KbOutMax=[]  KtOutMin=[]  KtOutMax=[]  IntegratorOutMin=[]  IntegratorOutMax=[]  FilterOutMin=[]  FilterOutMax=[]  SumI1OutMin=[]  SumI1OutMax=[]  SumI2OutMin=[]  SumI2OutMax=[]  SumI3OutMin=[]  SumI3OutMax=[]  SumDOutMin=[]  SumDOutMax=[]  DifferentiatorOutMin=[]  DifferentiatorOutMax=[]  FilterDiffOutCoefMin=[]  FilterDiffOutCoefMax=[]  ReciprocalOutMin=[]  ReciprocalOutMax=[]  SumDenOutMin=[]  SumDenOutMax=[]  SumNumOutMin=[]  SumNumOutMax=[]  DivideOutMin=[]  DivideOutMax=[]  IntegratorContinuousStateAttributes=''  IntegratorStateMustResolveToSignalObject=off  IntegratorRTWStateStorageClass=Auto  FilterContinuousStateAttributes=''  FilterStateMustResolveToSignalObject=off  FilterRTWStateStorageClass=Auto
  PID Controller1 : simulink/Continuous/PID Controller  Controller=PID  Form=Parallel  TimeDomain=Continuous-time  SampleTime=-1  IntegratorMethod=Forward Euler  ControllerParametersSource=internal  P=0  I=7  D=0  UseFilter=on  N=100  TunerSelectOption=Transfer Function Based (PID Tuner App)  InitialConditionSource=internal  InitialConditionForIntegrator=0  InitialConditionForFilter=0  DifferentiatorICPrevScaledInput=0  ExternalReset=none  TrackingMode=off  Kt=1  LimitOutput=off  UpperSaturationLimit=inf  LowerSaturationLimit=-inf  LinearizeAsGain=on  AntiWindupMode=none  Kb=1  POutMin=[]  POutMax=[]  IOutMin=[]  IOutMax=[]  DOutMin=[]  DOutMax=[]  NOutMin=[]  NOutMax=[]  SumOutMin=[]  SumOutMax=[]  SaturationOutMin=[]  SaturationOutMax=[]  PParamMin=[]  PParamMax=[]  IParamMin=[]  IParamMax=[]  DParamMin=[]  DParamMax=[]  NParamMin=[]  NParamMax=[]  KbParamMin=[]  KbParamMax=[]  KtParamMin=[]  KtParamMax=[]  KbOutMin=[]  KbOutMax=[]  KtOutMin=[]  KtOutMax=[]  IntegratorOutMin=[]  IntegratorOutMax=[]  FilterOutMin=[]  FilterOutMax=[]  SumI1OutMin=[]  SumI1OutMax=[]  SumI2OutMin=[]  SumI2OutMax=[]  SumI3OutMin=[]  SumI3OutMax=[]  SumDOutMin=[]  SumDOutMax=[]  DifferentiatorOutMin=[]  DifferentiatorOutMax=[]  FilterDiffOutCoefMin=[]  FilterDiffOutCoefMax=[]  ReciprocalOutMin=[]  ReciprocalOutMax=[]  SumDenOutMin=[]  SumDenOutMax=[]  SumNumOutMin=[]  SumNumOutMax=[]  DivideOutMin=[]  DivideOutMax=[]  IntegratorContinuousStateAttributes=''  IntegratorStateMustResolveToSignalObject=off  IntegratorRTWStateStorageClass=Auto  FilterContinuousStateAttributes=''  FilterStateMustResolveToSignalObject=off  FilterRTWStateStorageClass=Auto
  PWM Generator (DC-DC) : spsPWMGeneratorDCDCLib/PWM Generator (DC-DC)  Fsw=5000  Ts=0
  PWM Generator (DC-DC)1 : spsPWMGeneratorDCDCLib/PWM Generator (DC-DC)  Fsw=5000  Ts=0
  Series RLC Branch{,2..3,5} (4 alike) : spsSeriesRLCBranchLib/Series RLC Branch  LConnTagsString=__new0  RConnTagsString=__new0  BranchType=RC  Resistance=0.0001  Inductance=1e-3  SetiL0=off  InitialCurrent=0  Capacitance=1000e-6  Setx0=off  InitialVoltage=0  Measurements=None
  Series RLC Branch1 : spsSeriesRLCBranchLib/Series RLC Branch  LConnTagsString=__new0  RConnTagsString=__new0  BranchType=L  Resistance=0.0001  Inductance=1e-3  SetiL0=off  InitialCurrent=0  Capacitance=1000e-6  Setx0=off  InitialVoltage=0  Measurements=None
  Series RLC Branch4 : spsSeriesRLCBranchLib/Series RLC Branch  LConnTagsString=__new0  RConnTagsString=__new0  BranchType=L  Resistance=0.0001  Inductance=1e-3  SetiL0=off  InitialCurrent=0  Capacitance=1000e-6  Setx0=off  InitialVoltage=0  Measurements=None
  Sum : Sum  Inputs=|+-
  Sum1 : Sum  Inputs=|+-
  Voltage Measurement{,1..3} (4 alike) : spsVoltageMeasurementLib/Voltage Measurement  PhasorSimulation=off  OutputType=Complex  PSBequivalent=0
  charge_in + : PMIOPort  Side=Right
  charge_in - : PMIOPort  Port=2  Side=Right
  disch_out - : PMIOPort  Port=3  Side=Right
  disch_out + : PMIOPort  Port=4  Side=Right
  charge_out - : PMIOPort  Port=5  Side=Right
  charge_out + : PMIOPort  Port=6  Side=Right
  disch_in + : PMIOPort  Port=7  Side=Right
  disch_in - : PMIOPort  Port=8  Side=Right
  wires:
  [m1] -> Mosfet/1
  PWM Generator (DC-DC)/1 -> Display/1, [m11]
  PID Controller/1 -> PWM Generator (DC-DC)/1
  Constant1/1 -> Sum1/1
  PID Controller1/1 -> PWM Generator (DC-DC)1/1
  PWM Generator (DC-DC)1/1 -> Display1/1, [m12]
  Sum/1 -> PID Controller/1
  Constant/1 -> Sum/1
  [V12] -> Sum/2
  Sum1/1 -> PID Controller1/1
  [V11] -> Sum1/2
  [m2] -> Mosfet1/1
  [m12] -> Mosfet3/1
  [m11] -> Mosfet2/1
  Voltage Measurement/1 -> [V11]
  Voltage Measurement1/1 -> [V12]
  Voltage Measurement3/1 -> [V2]
  Voltage Measurement2/1 -> [V1]
  connections:
  disch_out +/RConn1 -- Voltage Measurement2/LConn1 -- Series RLC Branch/LConn1 -- Series RLC Branch1/RConn1
  disch_in -/RConn1 -- Voltage Measurement3/LConn2 -- Series RLC Branch2/RConn1 -- Mosfet/RConn1 -- Voltage Measurement2/LConn2 -- Series RLC Branch/RConn1 -- disch_out -/RConn1
  disch_in +/RConn1 -- Series RLC Branch2/LConn1 -- Voltage Measurement3/LConn1 -- Mosfet1/LConn1
  charge_out -/RConn1 -- Mosfet2/RConn1 -- Voltage Measurement/LConn2 -- Series RLC Branch3/RConn1 -- charge_in -/RConn1 -- Voltage Measurement1/LConn2 -- Series RLC Branch5/RConn1
  charge_out +/RConn1 -- Series RLC Branch5/LConn1 -- Voltage Measurement1/LConn1 -- Mosfet3/LConn1
  Mosfet1/RConn1 -- Series RLC Branch1/LConn1 -- Mosfet/LConn1
  Series RLC Branch4/LConn1 -- Mosfet2/LConn1 -- Mosfet3/RConn1
  Series RLC Branch3/LConn1 -- Voltage Measurement/LConn1 -- charge_in +/RConn1 -- Series RLC Branch4/RConn1

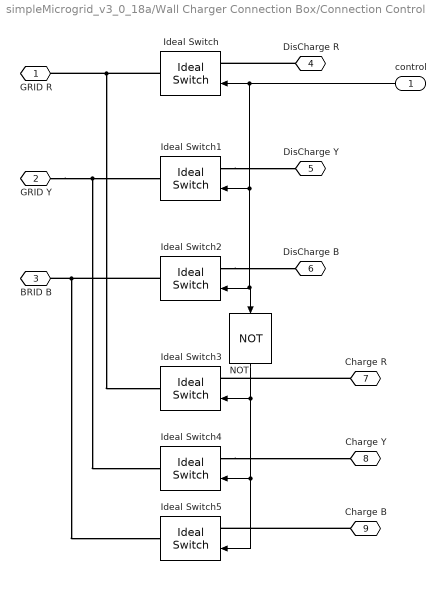
== system simpleMicrogrid_v3_0_18a/Wall Charger Connection Box/Connection Control ==
  control : Inport
  Ideal Switch{,1..5} (6 alike) : spsIdealSwitchLib/Ideal Switch  Ron=0.001  Lon=0  IC=0  Rs=1e5  Cs=inf  Measurements=off
  NOT : Logic  Operator=NOT  IconShape=distinctive  AllPortsSameDT=off  OutDataTypeStr=boolean
  GRID R : PMIOPort  Side=Left
  GRID Y : PMIOPort  Port=2  Side=Left
  BRID B : PMIOPort  Port=3  Side=Left
  DisCharge R : PMIOPort  Port=4  Side=Right
  DisCharge Y : PMIOPort  Port=5  Side=Right
  DisCharge B : PMIOPort  Port=6  Side=Right
  Charge R : PMIOPort  Port=7  Side=Right
  Charge Y : PMIOPort  Port=8  Side=Right
  Charge B : PMIOPort  Port=9  Side=Right
  wires:
  control/1 -> NOT/1, Ideal Switch2/1, Ideal Switch1/1, Ideal Switch/1
  NOT/1 -> Ideal Switch5/1, Ideal Switch4/1, Ideal Switch3/1
  connections:
  Ideal Switch/RConn1 -- Ideal Switch3/RConn1 -- GRID R/RConn1
  DisCharge R/RConn1 -- Ideal Switch/LConn1
  GRID Y/RConn1 -- Ideal Switch4/RConn1 -- Ideal Switch1/RConn1
  Ideal Switch1/LConn1 -- DisCharge Y/RConn1
  Ideal Switch2/LConn1 -- DisCharge B/RConn1
  Charge R/RConn1 -- Ideal Switch3/LConn1
  Ideal Switch2/RConn1 -- Ideal Switch5/RConn1 -- BRID B/RConn1
  Charge B/RConn1 -- Ideal Switch5/LConn1
  Ideal Switch4/LConn1 -- Charge Y/RConn1

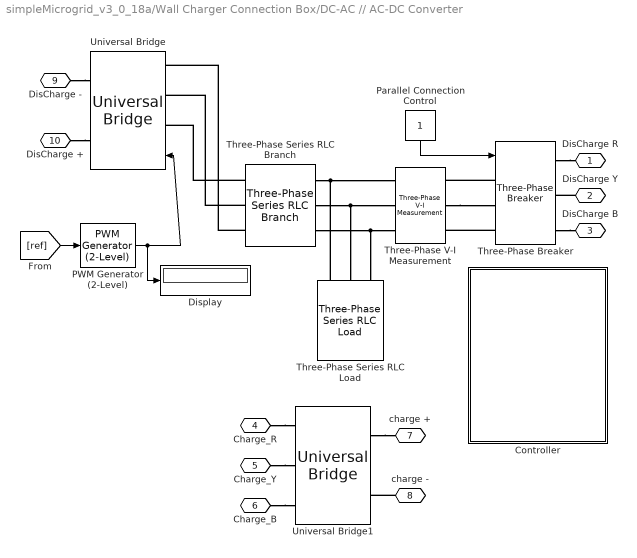
== system simpleMicrogrid_v3_0_18a/Wall Charger Connection Box/DC-AC // AC-DC Converter ==
  Controller : Subsystem
  Display : Display
  PWM Generator (2-Level) : spsPWMGenerator2LevelLib/PWM Generator (2-Level)  ModulatorType=Three-phase bridge (6 pulses)  ModulatorMode=Unsynchronized  Fc=4950  Pc=90  nF=27  MinMax="[ -1  1 ]"  SamplingTechnique=Natural  ModulatingSignals=off  m=0.8  Freq=60  Phase=0  Ts=2.02e-6  ShowCarrierOutport=off
  Parallel Connection Control : Constant
  Three-Phase Series RLC Branch : spsThreePhaseSeriesRLCBranchLib/Three-Phase Series RLC Branch  LConnTagsString=A|B|C  RConnTagsString=A|B|C  BranchType=RL  Resistance=0.004332  Inductance=0.0013789184  Capacitance=1e-6  Measurements=None
  Three-Phase Series RLC Load : spsThreePhaseSeriesRLCLoadLib/Three-Phase Series RLC Load  LConnTagsString=A|B|C  Configuration=Delta  NominalVoltage=380  Vabc=[1e3 1e3 1e3]  Vabcp=[1e3 1e3 1e3]  NominalFrequency=50  UnbalancedPower=off  ActivePower=100  InductivePower=0  CapacitivePower=5000  Pabc=[10e3 9e3 11e3]  QLabc=[100 90 110]  QCabc=[100 90 110]  Pabcp=[10e3 9e3 11e3]  QLabcp=[100 90 110]  QCabcp=[100 90 110]  Measurements=None  LoadType=constant Z
  Three-Phase V-I Measurement : spsThreePhaseVIMeasurementLib/Three-Phase V-I Measurement  VoltageMeasurement=phase-to-phase  SetLabelV=on  LabelV=Vabc_inv  Vpu=off  VpuLL=off  CurrentMeasurement=yes  SetLabelI=on  LabelI=Iabc_inv  Ipu=off  Pbase=100e6  Vbase=500e3  OutputType=Complex  PhasorSimulation=off  PSBequivalent=0
  Three-Phase Breaker : spsThreePhaseBreakerLib/Three-Phase Breaker  InitialState=open  SwitchA=on  SwitchB=on  SwitchC=on  SwitchTimes="[1/60  5/60]"  External=on  BreakerResistance=0.01  SnubberResistance=1e6  SnubberCapacitance=inf  Measurements=None
  Universal Bridge : spsUniversalBridgeLib/Universal Bridge  Arms=3  SnubberResistance=1e6  SnubberCapacitance=inf  Device=IGBT / Diodes  Ron=1e-3  Lon=0  ForwardVoltages=[0 0]  ForwardVoltage=0  GTOparameters=[ 10e-6 , 20e-6 ]  IGBTparameters=[ 1e-6 , 2e-6 ]  Measurements=None  Measurements_2=None  converterType=Rectifier
  Universal Bridge1 : spsUniversalBridgeLib/Universal Bridge  Arms=3  SnubberResistance=1e5  SnubberCapacitance=inf  Device=Diodes  Ron=1e-3  Lon=0  ForwardVoltages="[  0  0  ]"  ForwardVoltage=0  GTOparameters=[ 10e-6 , 20e-6 ]  IGBTparameters=[ 1e-6 , 2e-6 ]  Measurements=None  Measurements_2=None  converterType=Rectifier
  DisCharge R : PMIOPort  Side=Right
  DisCharge Y : PMIOPort  Port=2  Side=Right
  DisCharge B : PMIOPort  Port=3  Side=Right
  Charge_R : PMIOPort  Port=4  Side=Right
  Charge_Y : PMIOPort  Port=5  Side=Right
  Charge_B : PMIOPort  Port=6  Side=Right
  charge + : PMIOPort  Port=7  Side=Right
  charge - : PMIOPort  Port=8  Side=Right
  DisCharge - : PMIOPort  Port=9  Side=Right
  DisCharge + : PMIOPort  Port=10  Side=Right
  wires:
  PWM Generator (2-Level)/1 -> Display/1, Universal Bridge/1
  [ref] -> PWM Generator (2-Level)/1
  Parallel Connection Control/1 -> Three-Phase Breaker/1
  connections:
  DisCharge +/RConn1 -- Universal Bridge/RConn1
  DisCharge -/RConn1 -- Universal Bridge/RConn2
  Three-Phase Series RLC Branch/LConn1 -- Universal Bridge/LConn1
  Three-Phase Series RLC Branch/LConn2 -- Universal Bridge/LConn2
  Three-Phase Series RLC Branch/LConn3 -- Universal Bridge/LConn3
  Three-Phase Series RLC Branch/RConn1 -- Three-Phase V-I Measurement/LConn1 -- Three-Phase Series RLC Load/LConn1
  Three-Phase Series RLC Branch/RConn2 -- Three-Phase V-I Measurement/LConn2 -- Three-Phase Series RLC Load/LConn2
  Three-Phase Series RLC Branch/RConn3 -- Three-Phase V-I Measurement/LConn3 -- Three-Phase Series RLC Load/LConn3
  Three-Phase Breaker/LConn1 -- Three-Phase V-I Measurement/RConn1
  Three-Phase V-I Measurement/RConn2 -- Three-Phase Breaker/LConn2
  Three-Phase Breaker/LConn3 -- Three-Phase V-I Measurement/RConn3
  Three-Phase Breaker/RConn1 -- DisCharge R/RConn1
  DisCharge Y/RConn1 -- Three-Phase Breaker/RConn2
  Three-Phase Breaker/RConn3 -- DisCharge B/RConn1
  Charge_R/RConn1 -- Universal Bridge1/LConn1
  Charge_Y/RConn1 -- Universal Bridge1/LConn2
  Charge_B/RConn1 -- Universal Bridge1/LConn3
  charge -/RConn1 -- Universal Bridge1/RConn2
  Universal Bridge1/RConn1 -- charge +/RConn1

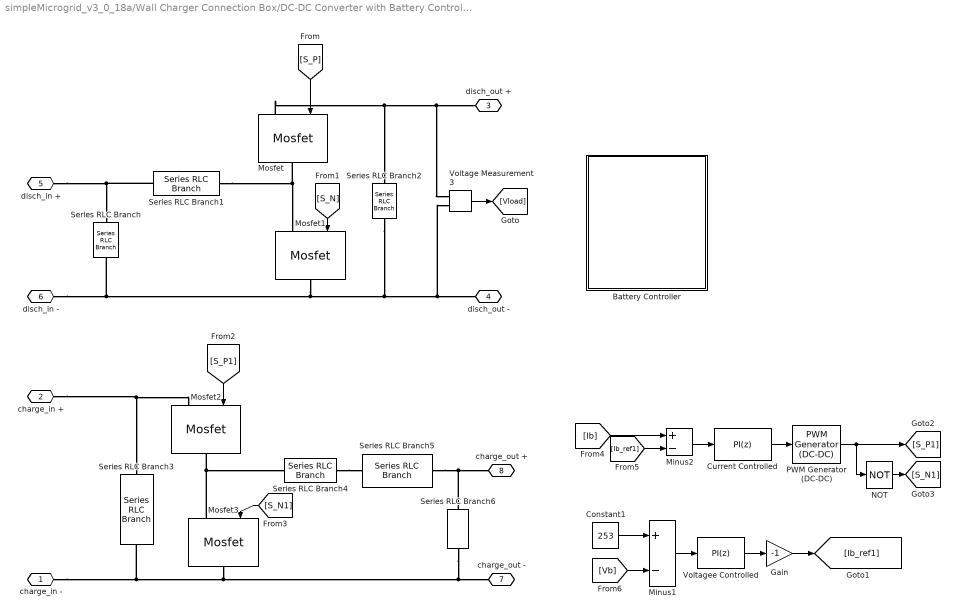
== system simpleMicrogrid_v3_0_18a/Wall Charger Connection Box/DC-DC Converter with Battery Controller ==
  Battery Controller : Subsystem
  Constant1 : Constant  Value=253
  Current Controlled : simulink/Continuous/PID Controller  Controller=PI  Form=Parallel  TimeDomain=Discrete-time  SampleTime=50e-6  IntegratorMethod=Forward Euler  ControllerParametersSource=internal  P=0.005  I=10  D=0  UseFilter=on  N=100  TunerSelectOption=Transfer Function Based (PID Tuner App)  InitialConditionSource=internal  InitialConditionForIntegrator=0.54  InitialConditionForFilter=0  DifferentiatorICPrevScaledInput=0  ExternalReset=none  TrackingMode=off  Kt=1  LimitOutput=on  UpperSaturationLimit=0.95  LowerSaturationLimit=0  LinearizeAsGain=off  AntiWindupMode=none  Kb=1  POutMin=[]  POutMax=[]  IOutMin=[]  IOutMax=[]  DOutMin=[]  DOutMax=[]  NOutMin=[]  NOutMax=[]  SumOutMin=[]  SumOutMax=[]  SaturationOutMin=[]  SaturationOutMax=[]  PParamMin=[]  PParamMax=[]  IParamMin=[]  IParamMax=[]  DParamMin=[]  DParamMax=[]  NParamMin=[]  NParamMax=[]  KbParamMin=[]  KbParamMax=[]  KtParamMin=[]  KtParamMax=[]  KbOutMin=[]  KbOutMax=[]  KtOutMin=[]  KtOutMax=[]  IntegratorOutMin=[]  IntegratorOutMax=[]  FilterOutMin=[]  FilterOutMax=[]  SumI1OutMin=[]  SumI1OutMax=[]  SumI2OutMin=[]  SumI2OutMax=[]  SumI3OutMin=[]  SumI3OutMax=[]  SumDOutMin=[]  SumDOutMax=[]  DifferentiatorOutMin=[]  DifferentiatorOutMax=[]  FilterDiffOutCoefMin=[]  FilterDiffOutCoefMax=[]  ReciprocalOutMin=[]  ReciprocalOutMax=[]  SumDenOutMin=[]  SumDenOutMax=[]  SumNumOutMin=[]  SumNumOutMax=[]  DivideOutMin=[]  DivideOutMax=[]  IntegratorContinuousStateAttributes=''  IntegratorStateMustResolveToSignalObject=off  IntegratorRTWStateStorageClass=Auto  FilterContinuousStateAttributes=''  FilterStateMustResolveToSignalObject=off  FilterRTWStateStorageClass=Auto
  Gain : Gain  Gain=-1
  Minus1 : Sum  Inputs=+-
  Minus2 : Sum  Inputs=+-
  Mosfet{,1..3} (4 alike) : spsMosfetLib/Mosfet  Ron=0.1  Lon=0  Rd=0.01  Vfd=0  IC=0  Rs=1e5  Cs=inf  Measurements=off
  NOT : Logic  Operator=NOT  IconShape=distinctive  AllPortsSameDT=off  OutDataTypeStr=boolean
  PWM Generator (DC-DC) : spsPWMGeneratorDCDCLib/PWM Generator (DC-DC)  Fsw=10e3  Ts=5e-6
  Series RLC Branch : spsSeriesRLCBranchLib/Series RLC Branch  LConnTagsString=__new0  RConnTagsString=__new0  BranchType=R  Resistance=10  Inductance=1e-3  SetiL0=off  InitialCurrent=0  Capacitance=1e-6  Setx0=off  InitialVoltage=0  Measurements=None
  Series RLC Branch1 : spsSeriesRLCBranchLib/Series RLC Branch  LConnTagsString=__new0  RConnTagsString=__new0  BranchType=RL  Resistance=0.05  Inductance=5.76e-4  SetiL0=off  InitialCurrent=0  Capacitance=1e-6  Setx0=off  InitialVoltage=0  Measurements=None
  Series RLC Branch2 : spsSeriesRLCBranchLib/Series RLC Branch  LConnTagsString=__new0  RConnTagsString=__new0  BranchType=RC  Resistance=0.001  Inductance=1e-3  SetiL0=off  InitialCurrent=0  Capacitance=1000e-6  Setx0=off  InitialVoltage=0  Measurements=None
  Series RLC Branch3 : spsSeriesRLCBranchLib/Series RLC Branch  LConnTagsString=__new0  RConnTagsString=__new0  BranchType=RC  Resistance=0.001  Inductance=1e-3  SetiL0=off  InitialCurrent=0  Capacitance=1000e-6  Setx0=off  InitialVoltage=0  Measurements=None
  Series RLC Branch4 : spsSeriesRLCBranchLib/Series RLC Branch  LConnTagsString=__new0  RConnTagsString=__new0  BranchType=RL  Resistance=0.05  Inductance=5.76e-4  SetiL0=off  InitialCurrent=0  Capacitance=1e-6  Setx0=off  InitialVoltage=0  Measurements=None
  Series RLC Branch5 : spsSeriesRLCBranchLib/Series RLC Branch  LConnTagsString=__new0  RConnTagsString=__new0  BranchType=R  Resistance=10  Inductance=1e-3  SetiL0=off  InitialCurrent=0  Capacitance=1e-6  Setx0=off  InitialVoltage=0  Measurements=None
  Series RLC Branch6 : spsSeriesRLCBranchLib/Series RLC Branch  LConnTagsString=__new0  RConnTagsString=__new0  BranchType=RC  Resistance=1e-3  Inductance=1e-3  SetiL0=off  InitialCurrent=0  Capacitance=5600e-6  Setx0=off  InitialVoltage=0  Measurements=None
  Voltage Measurement3 : spsVoltageMeasurementLib/Voltage Measurement  PhasorSimulation=off  OutputType=Complex  PSBequivalent=0
  Voltagee Controlled : simulink/Continuous/PID Controller  Controller=PI  Form=Parallel  TimeDomain=Discrete-time  SampleTime=50e-6  IntegratorMethod=Forward Euler  ControllerParametersSource=internal  P=40  I=2000  D=0  UseFilter=on  N=100  TunerSelectOption=Transfer Function Based (PID Tuner App)  InitialConditionSource=internal  InitialConditionForIntegrator=0  InitialConditionForFilter=0  DifferentiatorICPrevScaledInput=0  ExternalReset=none  TrackingMode=off  Kt=1  LimitOutput=on  UpperSaturationLimit=22  LowerSaturationLimit=0  LinearizeAsGain=off  AntiWindupMode=none  Kb=1  POutMin=[]  POutMax=[]  IOutMin=[]  IOutMax=[]  DOutMin=[]  DOutMax=[]  NOutMin=[]  NOutMax=[]  SumOutMin=[]  SumOutMax=[]  SaturationOutMin=[]  SaturationOutMax=[]  PParamMin=[]  PParamMax=[]  IParamMin=[]  IParamMax=[]  DParamMin=[]  DParamMax=[]  NParamMin=[]  NParamMax=[]  KbParamMin=[]  KbParamMax=[]  KtParamMin=[]  KtParamMax=[]  KbOutMin=[]  KbOutMax=[]  KtOutMin=[]  KtOutMax=[]  IntegratorOutMin=[]  IntegratorOutMax=[]  FilterOutMin=[]  FilterOutMax=[]  SumI1OutMin=[]  SumI1OutMax=[]  SumI2OutMin=[]  SumI2OutMax=[]  SumI3OutMin=[]  SumI3OutMax=[]  SumDOutMin=[]  SumDOutMax=[]  DifferentiatorOutMin=[]  DifferentiatorOutMax=[]  FilterDiffOutCoefMin=[]  FilterDiffOutCoefMax=[]  ReciprocalOutMin=[]  ReciprocalOutMax=[]  SumDenOutMin=[]  SumDenOutMax=[]  SumNumOutMin=[]  SumNumOutMax=[]  DivideOutMin=[]  DivideOutMax=[]  IntegratorContinuousStateAttributes=''  IntegratorStateMustResolveToSignalObject=off  IntegratorRTWStateStorageClass=Auto  FilterContinuousStateAttributes=''  FilterStateMustResolveToSignalObject=off  FilterRTWStateStorageClass=Auto
  charge_in - : PMIOPort  Side=Left
  charge_in + : PMIOPort  Port=2  Side=Left
  disch_out + : PMIOPort  Port=3  Side=Right
  disch_out - : PMIOPort  Port=4  Side=Right
  disch_in + : PMIOPort  Port=5  Side=Right
  disch_in - : PMIOPort  Port=6  Side=Right
  charge_out - : PMIOPort  Port=7  Side=Right
  charge_out + : PMIOPort  Port=8  Side=Right
  wires:
  [S_P] -> Mosfet/1
  [S_N] -> Mosfet1/1
  Voltage Measurement3/1 -> [Vload]
  [S_P1] -> Mosfet2/1
  [S_N1] -> Mosfet3/1
  Current Controlled/1 -> PWM Generator (DC-DC)/1
  NOT/1 -> [S_N1]
  [Ib] -> Minus2/1
  Minus2/1 -> Current Controlled/1
  [Ib_ref1] -> Minus2/2
  PWM Generator (DC-DC)/1 -> NOT/1, [S_P1]
  Voltagee Controlled/1 -> Gain/1
  Minus1/1 -> Voltagee Controlled/1
  Gain/1 -> [Ib_ref1]
  Constant1/1 -> Minus1/1
  [Vb] -> Minus1/2
  connections:
  disch_in +/RConn1 -- Series RLC Branch1/LConn1 -- Series RLC Branch/LConn1
  disch_in -/RConn1 -- Mosfet1/RConn1 -- Series RLC Branch2/RConn1 -- Voltage Measurement3/LConn2 -- disch_out -/RConn1 -- Series RLC Branch/RConn1
  Series RLC Branch1/RConn1 -- Mosfet1/LConn1 -- Mosfet/RConn1
  Mosfet/LConn1 -- Series RLC Branch2/LConn1 -- Voltage Measurement3/LConn1 -- disch_out +/RConn1
  charge_in +/RConn1 -- Mosfet2/LConn1 -- Series RLC Branch3/LConn1
  charge_in -/RConn1 -- Mosfet3/RConn1 -- Series RLC Branch6/RConn1 -- charge_out -/RConn1 -- Series RLC Branch3/RConn1
  Mosfet3/LConn1 -- Mosfet2/RConn1 -- Series RLC Branch4/LConn1
  Series RLC Branch4/RConn1 -- Series RLC Branch5/RConn1
  Series RLC Branch5/LConn1 -- Series RLC Branch6/LConn1 -- charge_out +/RConn1

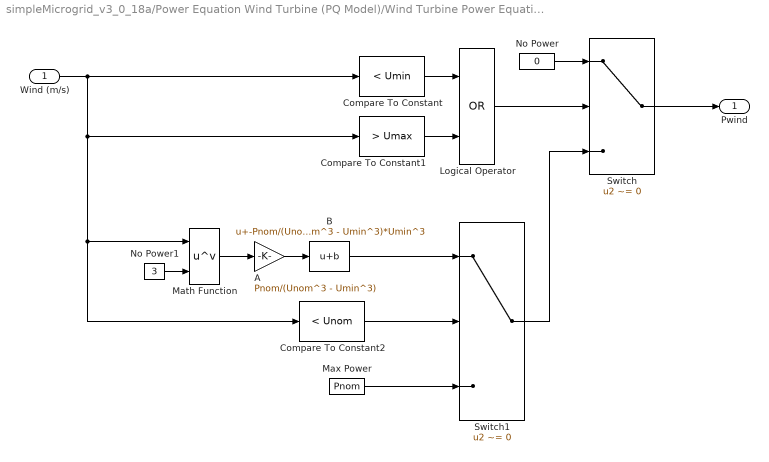
== system simpleMicrogrid_v3_0_18a/Power Equation Wind Turbine (PQ Model)/Wind Turbine Power Equation/Cubic Power with Cutoff ==
  Wind (m/s) : Inport
  A : Gain  Gain=Pnom/(Unom^3 - Umin^3)
  B : Bias  Bias=-Pnom/(Unom^3 - Umin^3)*Umin^3
  Compare To Constant : simulink/Logic and Bit Operations/Compare To Constant  relop=<  const=Umin  OutDataTypeStr=boolean
  Compare To Constant1 : simulink/Logic and Bit Operations/Compare To Constant  relop=>  const=Umax  OutDataTypeStr=boolean
  Compare To Constant2 : simulink/Logic and Bit Operations/Compare To Constant  relop=<  const=Unom  OutDataTypeStr=boolean
  Logical Operator : Logic  Operator=OR  AllPortsSameDT=off  OutDataTypeStr=boolean
  Math Function : Math  Operator=pow  SaturateOnIntegerOverflow=on
  Max Power : Constant  Value=Pnom
  No Power : Constant  Value=0
  No Power1 : Constant  Value=3
  Switch : Switch  Criteria=u2 ~= 0  ZeroCross=off
  Switch1 : Switch  Criteria=u2 ~= 0  ZeroCross=off
  Pwind : Outport  VectorParamsAs1DForOutWhenUnconnected=off
  wires:
  B/1 -> Switch1/1
  Compare To Constant2/1 -> Switch1/2
  Compare To Constant1/1 -> Logical Operator/2
  Math Function/1 -> A/1
  No Power1/1 -> Math Function/2
  No Power/1 -> Switch/1
  Switch1/1 -> Switch/3
  Max Power/1 -> Switch1/3
  Wind (m/s)/1 -> Compare To Constant/1, Compare To Constant1/1, Math Function/1, Compare To Constant2/1
  A/1 -> B/1
  Logical Operator/1 -> Switch/2
  Switch/1 -> Pwind/1
  Compare To Constant/1 -> Logical Operator/1

== system simpleMicrogrid_v3_0_18a/Power Equation Wind Turbine (PQ Model)/Wind Turbine Power Equation/Wind Turbine Properties ==
  Wind (m/s) : Inport
  Compare To Constant : simulink/Logic and Bit Operations/Compare To Constant  relop=<  const=Umin  OutDataTypeStr=boolean
  Compare To Constant1 : simulink/Logic and Bit Operations/Compare To Constant  relop=>  const=Umax  OutDataTypeStr=boolean
  Compare To Constant2 : simulink/Logic and Bit Operations/Compare To Constant  relop=<  const=Unom  OutDataTypeStr=boolean
  Logical Operator : Logic  Operator=OR  AllPortsSameDT=off  OutDataTypeStr=boolean
  Max Power : Constant  Value=Pnom
  No Power : Constant  Value=0
  Properties : Subsystem
  Switch : Switch  Criteria=u2 ~= 0  ZeroCross=off
  Switch1 : Switch  Criteria=u2 ~= 0  ZeroCross=off
  Pwind : Outport  VectorParamsAs1DForOutWhenUnconnected=off
  wires:
  Compare To Constant/1 -> Logical Operator/1
  Switch/1 -> Pwind/1
  Logical Operator/1 -> Switch/2
  Wind (m/s)/1 -> Compare To Constant2/1, Properties/1(In1), Compare To Constant1/1, Compare To Constant/1
  Max Power/1 -> Switch1/3
  Switch1/1 -> Switch/3
  No Power/1 -> Switch/1
  Compare To Constant1/1 -> Logical Operator/2
  Compare To Constant2/1 -> Switch1/2
  Properties/1(Out1) -> Switch1/1

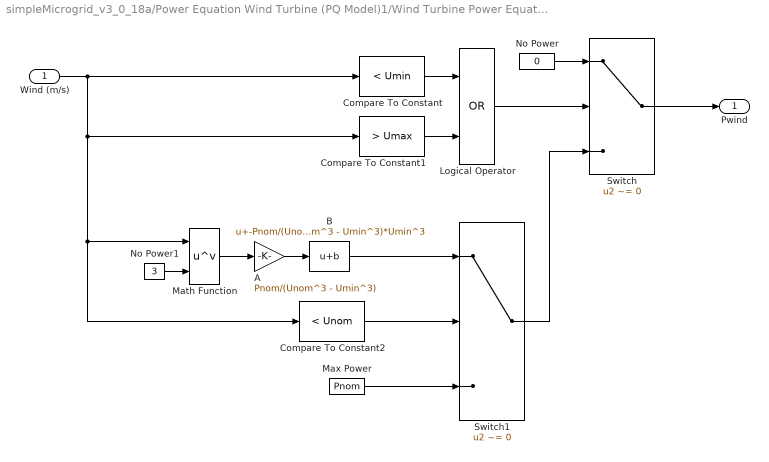
== system simpleMicrogrid_v3_0_18a/Power Equation Wind Turbine (PQ Model)1/Wind Turbine Power Equation/Cubic Power with Cutoff ==
  Wind (m/s) : Inport
  A : Gain  Gain=Pnom/(Unom^3 - Umin^3)
  B : Bias  Bias=-Pnom/(Unom^3 - Umin^3)*Umin^3
  Compare To Constant : simulink/Logic and Bit Operations/Compare To Constant  relop=<  const=Umin  OutDataTypeStr=boolean
  Compare To Constant1 : simulink/Logic and Bit Operations/Compare To Constant  relop=>  const=Umax  OutDataTypeStr=boolean
  Compare To Constant2 : simulink/Logic and Bit Operations/Compare To Constant  relop=<  const=Unom  OutDataTypeStr=boolean
  Logical Operator : Logic  Operator=OR  AllPortsSameDT=off  OutDataTypeStr=boolean
  Math Function : Math  Operator=pow  SaturateOnIntegerOverflow=on
  Max Power : Constant  Value=Pnom
  No Power : Constant  Value=0
  No Power1 : Constant  Value=3
  Switch : Switch  Criteria=u2 ~= 0  ZeroCross=off
  Switch1 : Switch  Criteria=u2 ~= 0  ZeroCross=off
  Pwind : Outport  VectorParamsAs1DForOutWhenUnconnected=off
  wires:
  B/1 -> Switch1/1
  Compare To Constant2/1 -> Switch1/2
  Compare To Constant1/1 -> Logical Operator/2
  Math Function/1 -> A/1
  No Power1/1 -> Math Function/2
  No Power/1 -> Switch/1
  Switch1/1 -> Switch/3
  Max Power/1 -> Switch1/3
  Wind (m/s)/1 -> Compare To Constant/1, Compare To Constant1/1, Math Function/1, Compare To Constant2/1
  A/1 -> B/1
  Logical Operator/1 -> Switch/2
  Switch/1 -> Pwind/1
  Compare To Constant/1 -> Logical Operator/1
